simulink model "sogi_pll_validation"  (R2025b)
settings: Solver=FixedStepDiscrete  StartTime=0.0  StopTime=T_pll_sim  FixedStep=T_pll  RelTol=1e-3
settings Model: Creator=hemanggadhvi  LastModifiedBy=hemanggadhvi

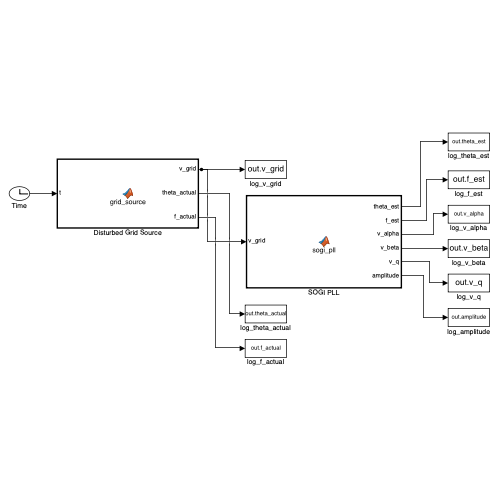
[thumbnail: Simulink's stored preview of the top-level diagram]
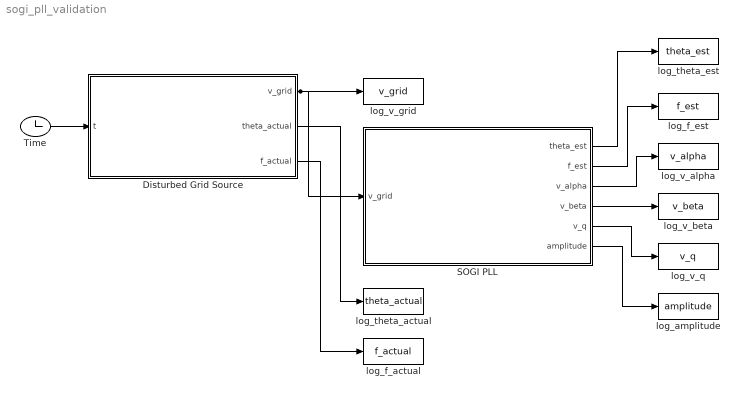
== system sogi_pll_validation ==
  Disturbed Grid Source : MATLAB Function  TreatAsAtomicUnit=on
  SOGI PLL : MATLAB Function  TreatAsAtomicUnit=on
  Time : Clock
  log_amplitude : ToWorkspace  VariableName=amplitude  SaveFormat=Timeseries  SampleTime=-1
  log_f_actual : ToWorkspace  VariableName=f_actual  SaveFormat=Timeseries  SampleTime=-1
  log_f_est : ToWorkspace  VariableName=f_est  SaveFormat=Timeseries  SampleTime=-1
  log_theta_actual : ToWorkspace  VariableName=theta_actual  SaveFormat=Timeseries  SampleTime=-1
  log_theta_est : ToWorkspace  VariableName=theta_est  SaveFormat=Timeseries  SampleTime=-1
  log_v_alpha : ToWorkspace  VariableName=v_alpha  SaveFormat=Timeseries  SampleTime=-1
  log_v_beta : ToWorkspace  VariableName=v_beta  SaveFormat=Timeseries  SampleTime=-1
  log_v_grid : ToWorkspace  VariableName=v_grid  SaveFormat=Timeseries  SampleTime=-1
  log_v_q : ToWorkspace  VariableName=v_q  SaveFormat=Timeseries  SampleTime=-1
  wires:
  SOGI PLL/3(v_alpha) -> log_v_alpha/1
  SOGI PLL/2(f_est) -> log_f_est/1
  Disturbed Grid Source/3(f_actual) -> log_f_actual/1
  SOGI PLL/5(v_q) -> log_v_q/1
  SOGI PLL/1(theta_est) -> log_theta_est/1
  Disturbed Grid Source/2(theta_actual) -> log_theta_actual/1
  SOGI PLL/4(v_beta) -> log_v_beta/1
  Disturbed Grid Source/1(v_grid) -> log_v_grid/1, SOGI PLL/1(v_grid)
  SOGI PLL/6(amplitude) -> log_amplitude/1
  Time/1 -> Disturbed Grid Source/1(t)

== matlab function sogi_pll_validation/SOGI PLL ==
  data: v_grid input; theta_est output; f_est output; v_alpha output; v_beta output; v_q output; amplitude output
function [theta_est,f_est,v_alpha,v_beta,v_q,amplitude] = sogi_pll(v_grid)
%#codegen
persistent va vb theta omega integ
if isempty(va); va=0; vb=0; theta=0; omega=2*pi*50; integ=0; end
Ts=5.0000000000000002e-05; k=1.4142135623730951; kp=106.61308829222321; ki=5684.8921350274704; wmin=2*pi*45; wmax=2*pi*55;
dva1=k*omega*(v_grid-va)-omega*vb; dvb1=omega*va;
va_p=va+Ts*dva1; vb_p=vb+Ts*dvb1;
dva2=k*omega*(v_grid-va_p)-omega*vb_p; dvb2=omega*va_p;
va=va+0.5*Ts*(dva1+dva2); vb=vb+0.5*Ts*(dvb1+dvb2);
amplitude=sqrt(va*va+vb*vb); norm_amp=max(amplitude,0.1*40.799999999999997);
vq=(va*cos(theta)+vb*sin(theta))/norm_amp;
unsat=2*pi*50+kp*vq+integ; omega=min(max(unsat,wmin),wmax);
if (unsat==omega) || (unsat>wmax && vq<0) || (unsat<wmin && vq>0); integ=integ+Ts*ki*vq; end
theta=mod(theta+Ts*omega,2*pi);
theta_est=theta; f_est=omega/(2*pi); v_alpha=va; v_beta=vb; v_q=vq;
end

== matlab function sogi_pll_validation/Disturbed Grid Source ==
  data: t input; v_grid output; theta_actual output; f_actual output
function [v_grid,theta_actual,f_actual] = grid_source(t)
f0=50; f1=52; ts=0.12; tj=0.22; jump=0.3490658503988659;
if t < ts; f_actual=f0; theta=2*pi*f0*t; else; f_actual=f1; theta=2*pi*f0*ts+2*pi*f1*(t-ts); end
if t >= tj; theta=theta+jump; end
if t >= 0.29999999999999999 && t < 0.35999999999999999; envelope=0.69999999999999996; else; envelope=1; end
v_grid=40.799999999999997*envelope*(sin(theta)+0.029999999999999999*sin(5*theta)+0.02*sin(7*theta)+0.002*sin(2*pi*1300*t));
theta_actual=mod(theta,2*pi);
end
